simulink model "Malha_Aberta_Malha_Fechada"  (Simulink 8.1)
settings: Solver=ode45  StartTime=0.0  StopTime=200  MaxStep=0.01  RelTol=1e-9
settings Model: Creator=deniseehector  LastModifiedBy=hector
settings OptimizationCC: InitFltsAndDblsToZero=on
settings DebuggingCC: StrictBusMsg=Warning

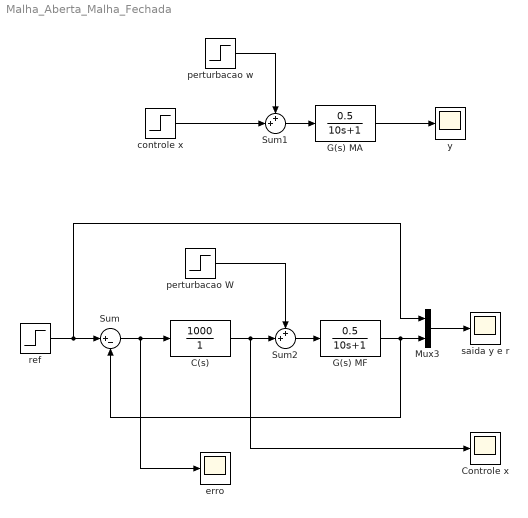
== system Malha_Aberta_Malha_Fechada ==
  C(s) : TransferFcn  Numerator=[1000]  Denominator=[1]
  Controle x : Scope
      settings: SaveName=ScopeData2
  G(s) MA : TransferFcn  Numerator=[0.5]  Denominator=[10 1]
  G(s) MF : TransferFcn  Numerator=[0.5]  Denominator=[10 1]
  Mux3 : Mux  Inputs=2
  Sum : Sum  Inputs=|+-
  Sum1 : Sum  Inputs=++|
  Sum2 : Sum  Inputs=++|
  controle x : Step  Time=0  SampleTime=0
  "erro " : Scope
      settings: SaveName=ScopeData3
  perturbacao W : Step  Time=100  After=0.5  SampleTime=0
  perturbacao w : Step  Time=100  After=0.25  SampleTime=0
  ref : Step  Time=0  SampleTime=0
  saida y e r : Scope
  y : Scope
  wires:
  Mux3/1 -> saida y e r/1
  ref/1 -> Sum/1, Mux3/1
  Sum/1 -> C(s)/1, "erro "/1
  G(s) MF/1 -> Sum/2, Mux3/2
  C(s)/1 -> Controle x/1, Sum2/2
  G(s) MA/1 -> y/1
  controle x/1 -> Sum1/2
  Sum1/1 -> G(s) MA/1
  perturbacao w/1 -> Sum1/1
  Sum2/1 -> G(s) MF/1
  perturbacao W/1 -> Sum2/1
